simulink model "soc_fmcw_proc"  (R2025b)
settings: Solver=FixedStepDiscrete  StartTime=0.0  StopTime=10.0  RelTol=1e-3  EnableMultiTasking=on
settings Model: Creator=kimsteph  LastModifiedBy=kimsteph
settings SolverCC: PositivePriorityOrder=on
settings OptimizationCC: DefaultParameterBehavior=Inlined  EnhancedBackFolding=on  PassReuseOutputArgsAs=Individual arguments  ZeroExternalMemoryAtStartup=off  ZeroInternalMemoryAtStartup=off  MaxStackSize=64  OptimizeBlockOrder=speed  DifferentSizesBufferReuse=on  OptimizationCustomize=off  EfficientTunableParamExpr=on
settings DebuggingCC: ParameterTunabilityLossMsg=error
settings HardwareCC: ProdBitPerLong=64.0  ProdLargestAtomicInteger=LongLong  ProdLargestAtomicFloat=Double  ProdLongLongMode=on  ProdHWDeviceType=ARM Compatible->ARM Cortex-A (64-bit)  HardwareBoardFeatureSet=SoCBlockset
settings ModelReferenceCC: ModelReferenceNumInstancesAllowed=Single
settings SFSimCC: MATLABDynamicMemAlloc=off
settings RTWCC: SystemTargetFile=ert.tlc  HardwareBoard=Xilinx Zynq UltraScale+ RFSoC ZCU111 Evaluation Kit  TLCOptions="-aInlineSetEventsForThisBaseRateFcn=TLC_FALSE -aSuppressMultiTaskScheduler=TLC_FALSE  -aRateBasedStepFcn=0"  TemplateMakefile=ert_default_tmf  Toolchain=Linaro AArch64 Linux v6.3.1  Description=Embedded Coder
settings CodeAppCC: ForceParamTrailComments=on  IgnoreCustomStorageClasses=off  OperatorAnnotations=on  SimulinkDataObjDesc=on  SFDataObjDesc=on  InsertBlockDesc=on
settings ERTTargetCC: SubcomponentCodeInterfacePackaging=Nonreusable function

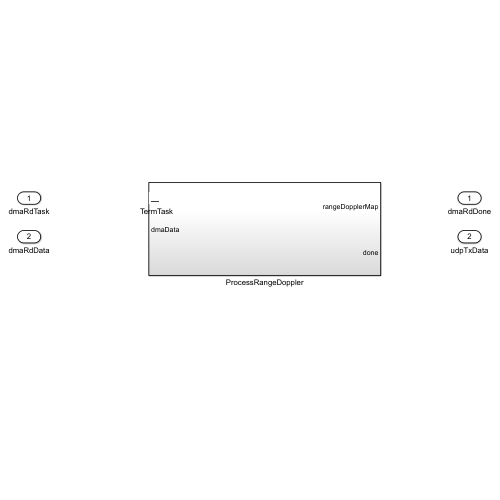
[thumbnail: Simulink's stored preview of the top-level diagram]
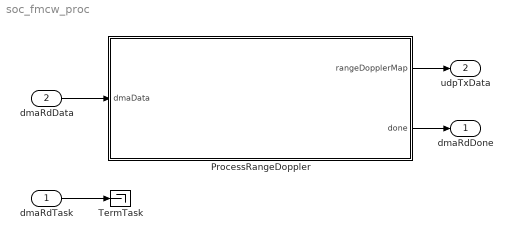
== system soc_fmcw_proc ==
  dmaRdTask : Inport
  dmaRdData : Inport  Port=2
  ProcessRangeDoppler : Subsystem
  TermTask : Terminator
  dmaRdDone : Outport
  udpTxData : Outport  Port=2
  wires:
  dmaRdData/1 -> ProcessRangeDoppler/1(dmaData)
  dmaRdTask/1 -> TermTask/1
  ProcessRangeDoppler/2(done) -> dmaRdDone/1
  ProcessRangeDoppler/1(rangeDopplerMap) -> udpTxData/1

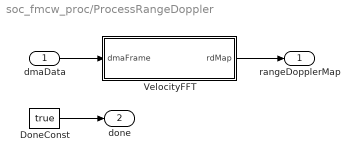
== system soc_fmcw_proc/ProcessRangeDoppler ==
  dmaData : Inport
  DoneConst : Constant  Value=true  OutDataTypeStr=boolean
  VelocityFFT : MATLAB Function  TreatAsAtomicUnit=on
  rangeDopplerMap : Outport
  done : Outport  Port=2
  wires:
  dmaData/1 -> VelocityFFT/1(dmaFrame)
  DoneConst/1 -> done/1
  VelocityFFT/1(rdMap) -> rangeDopplerMap/1

== matlab function soc_fmcw_proc/ProcessRangeDoppler/VelocityFFT ==
  data: dmaFrame input; rdMap output
function rdMap = VelocityFFT(dmaFrame)
% Velocity FFT for FMCW radar
% Input: dmaFrame (1D vector, N_range*N_chirps elements)
% Output: rdMap (N_range x N_chirps Range-Doppler map)

N_range = uint32(1024);
N_chirps = uint32(256);

% Reshape to Range x Chirp matrix
cpiMatrix = reshape(dmaFrame, [N_range, N_chirps]);

% Velocity FFT along chirp dimension
rdMap = fft(cpiMatrix, double(N_chirps), 2);

% Take magnitude squared
rdMap = abs(rdMap).^2;
